simulink model "mage2017_feedback_PKmodel"  (R2016a)
settings: Solver=ode15s  StartTime=0.0  StopTime=3000  RelTol=1e-3
undefined symbols (not defined in the file or in its folder): sigbuilder_block
libraries: simulink x2, simulink_extras x1
settings Model: Creator=bscottferguson  LastModifiedBy=petermage
settings DataIOCC: SaveFormat=StructureWithTime  SaveOutput=off  SaveTime=off
settings OptimizationCC: ExpressionDepthLimit=2147483647
settings DebuggingCC: UnderspecifiedInitializationDetection=Classic  MergeDetectMultiDrivingBlocksExec=none  SolverPrmCheckMsg=warning  AllowSymbolicDim=off  StateNameClashWarn=warning
settings HardwareCC: ProdBitPerPointer=32  ProdLargestAtomicFloat=None  ProdIntDivRoundTo=Undefined  ProdEndianess=Unspecified  ProdWordSize=32  ProdHWDeviceType=32-bit Generic
settings ModelReferenceCC: PropagateSignalLabelsOutOfModel=off
settings ConfigComp: CovModelRefEnable=Off

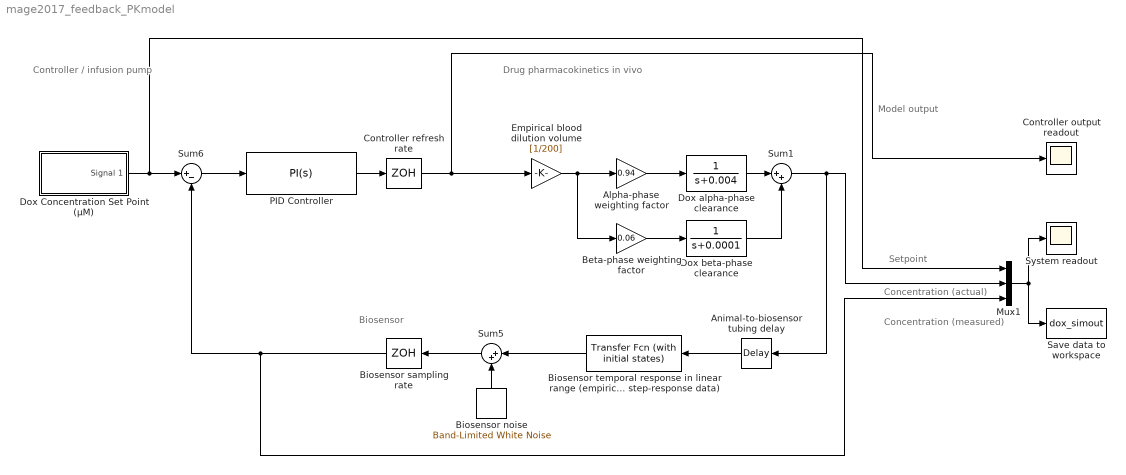
== system mage2017_feedback_PKmodel ==
  note: Model output
  note: Biosensor
  note: Drug pharmacokinetics in vivo
  note: Controller /
      | infusion pump
  note: Setpoint
  note: Concentration (actual)
  note: Concentration (measured)
  Alpha-phase weighting factor : Gain  Gain=0.94
  Animal-to-biosensor tubing delay : TransportDelay  DelayTime=40
  Beta-phase weighting factor : Gain  Gain=0.06
  Biosensor noise : simulink/Sources/Band-Limited White Noise  Cov=[0.00002]  Ts=.1  seed=[23341]
  "Biosensor sampling rate " : ZeroOrderHold  SampleTime=11
  "Biosensor temporal response in linear range (empirical, from step-response data)" : simulink_extras/Additional Linear/Transfer Fcn (with initial states)  N=0.0229  D=[1 0.02217]  X0=7e-4
  Controller refresh rate : ZeroOrderHold  SampleTime=5
  Controller output readout : Scope
  Dox Concentration Set Point (µM) : Subsystem  Tag=STV Subsys  LoadFcn=sigbuilder_block('load');  StartFcn=sigbuilder_block('start');  StopFcn=sigbuilder_block('stop');  ClipboardFcn=sigbuilder_block('clipboard');  mask(Sigbuilder block){}
      mask help: Simulink:masks:SigbuilderBlock_MD
      mask init:
      | if ~strcmp(get_param(bdroot(gcbh),'SimulationStatus'),'stopped') tuvar = sigbuilder_block('maskInit'); end
      settings: CopyFcn=sigbuilder_block('copy');  DeleteFcn=sigbuilder_block('delete');  ModelCloseFcn=sigbuilder_block('modelClose');  PreSaveFcn=sigbuilder_block('preSave');  PauseFcn=sigbuilder_block('pause');  ContinueFcn=sigbuilder_block('continue');  NameChangeFcn=sigbuilder_block('namechange');  OpenFcn=sigbuilder_block('open',[125.901 202.84 1110.13 399.685 ]);  CloseFcn=sigbuilder_block('close');
      mask Display: plot(0, 0, 100, 100,[2, 2, 32, 32, 2], [68, 8, 8, 68, 68],[32, 2], [38, 38], [32, 19, 2],[53, 60, 44], [32, 17, 17, 2],[16, 16, 31, 31]);txt = getActiveGroup(gcbh);text(2, 100, txt,'verticalAlignment', 'top');
  Dox alpha-phase clearance : TransferFcn  Denominator=[1 0.004]
  Dox beta-phase clearance : TransferFcn  Denominator=[1 0.0001]
  Empirical blood dilution volume : Gain  Gain=[1/200]
  Mux1 : Mux  Inputs=3
  PID Controller : simulink/Continuous/PID Controller  Controller=PI  TimeDomain=Continuous-time  SampleTime=-1  IntegratorMethod=Forward Euler  FilterMethod=Backward Euler  Form=Parallel  UseFilter=on  ControllerParametersSource=internal  P=0.99  I=0.0035  D=31.5143505390179  N=0.0502328378036205  InitialConditionSource=internal  InitialConditionForIntegrator=1e-5  InitialConditionForFilter=1e-5  ExternalReset=none  LimitOutput=on  UpperSaturationLimit=10  LowerSaturationLimit=0  LinearizeAsGain=off  AntiWindupMode=none  Kb=1  TrackingMode=off  Kt=1  PParamMin=[]  PParamMax=[]  IParamMin=[]  IParamMax=[]  DParamMin=[]  DParamMax=[]  NParamMin=[]  NParamMax=[]  KbParamMin=[]  KbParamMax=[]  KtParamMin=[]  KtParamMax=[]  POutMin=[]  POutMax=[]  IOutMin=[]  IOutMax=[]  DOutMin=[]  DOutMax=[]  NOutMin=[]  NOutMax=[]  KbOutMin=[]  KbOutMax=[]  KtOutMin=[]  KtOutMax=[]  IntegratorOutMin=[]  IntegratorOutMax=[]  FilterOutMin=[]  FilterOutMax=[]  SumOutMin=[]  SumOutMax=[]  SumI1OutMin=[]  SumI1OutMax=[]  SumI2OutMin=[]  SumI2OutMax=[]  SumI3OutMin=[]  SumI3OutMax=[]  SumDOutMin=[]  SumDOutMax=[]  SaturationOutMin=[]  SaturationOutMax=[]  IntegratorContinuousStateAttributes=''  IntegratorStateMustResolveToSignalObject=off  IntegratorRTWStateStorageClass=Auto  FilterContinuousStateAttributes=''  FilterStateMustResolveToSignalObject=off  FilterRTWStateStorageClass=Auto  DifferentiatorICPrevScaledInput=0  DifferentiatorOutMin=[]  DifferentiatorOutMax=[]
  Save data to workspace : ToWorkspace  VariableName=dox_simout  SampleTime=1
  Sum1 : Sum  Inputs=|++
  Sum5 : Sum  Inputs=|++
  Sum6 : Sum  Inputs=|+-
  System readout : Scope
  wires:
  Mux1/1 -> System readout/1, Save data to workspace/1
  Sum6/1 -> PID Controller/1
  Biosensor noise/1 -> Sum5/2
  Dox beta-phase clearance/1 -> Sum1/2
  Dox Concentration Set Point (µM)/1(Signal 1) -> Mux1/1, Sum6/1
  Dox alpha-phase clearance/1 -> Sum1/1
  "Biosensor temporal response in linear range (empirical, from step-response data)"/1 -> Sum5/1
  Alpha-phase weighting factor/1 -> Dox alpha-phase clearance/1
  Beta-phase weighting factor/1 -> Dox beta-phase clearance/1
  Sum5/1 -> "Biosensor sampling rate "/1
  Controller refresh rate/1 -> Empirical blood dilution volume/1, Controller output readout/1
  PID Controller/1 -> Controller refresh rate/1
  Empirical blood dilution volume/1 -> Alpha-phase weighting factor/1, Beta-phase weighting factor/1
  Animal-to-biosensor tubing delay/1 -> "Biosensor temporal response in linear range (empirical, from step-response data)"/1
  Sum1/1 -> Mux1/2, Animal-to-biosensor tubing delay/1
  "Biosensor sampling rate "/1 -> Mux1/3, Sum6/2

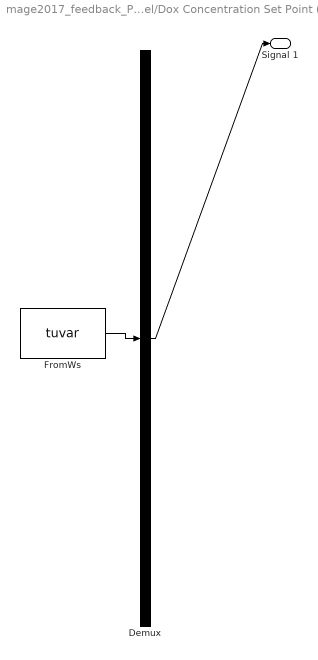
== system mage2017_feedback_PKmodel/Dox Concentration Set Point (µM) ==
  Demux : Demux  Tag=STV Demux  Outputs=1
  FromWs : FromWorkspace  Tag=STV FromWs  VariableName=tuvar  SampleTime=0
      SigBuilderData=|
      | common.afterFinalStr = 'Extrapolate'
      | common.sampleTime = 0
      | dataSet.timeRange = [-1000 9000]
      | dataSet.name = 'Group 1'
      | sbobj.Groups.Name = 'Group 1'
      | sbobj.Groups.Signals.Name = 'Signal 1'
      | sbobj.Groups.Signals.XData = [-1000 235 235 7200 7200 9000]
      | sbobj.Groups.Signals.YData = [0 0 0.646 0.646 0 0]
      | sbobj.Groups.TimeRange = [-1000 9000]
  Signal 1 : Outport  Tag=STV Outport
  wires:
  FromWs/1 -> Demux/1
  Demux/1 -> Signal 1/1
